simulink model "regcontrol_model"  (Simulink 9.1)
settings: Solver=VariableStepAuto  StartTime=0.0  StopTime=10.0  RelTol=1e-3
values from neighbouring files (symbols this model uses):
  BandWidth = Simulink.Parameter    [start.m]
  BaseVoltage = Simulink.Parameter    [start.m]
  CogenEnabled = false    [regcontrol_emulator.m]    (also in start.m = Simulink.Parameter)
  IsReversible = Simulink.Parameter    [start.m]
  LDC_Z = Simulink.Parameter    [start.m]
  PTratio = Simulink.Parameter    [start.m]
  RevBand = Simulink.Parameter    [start.m]
  RevVreg = Simulink.Parameter    [start.m]
  TapLimitPerChange = Simulink.Parameter    [start.m]
  UsingRegulatedBus = Simulink.Parameter    [start.m]
  Vlimit = Simulink.Parameter    [start.m]
  Vreg = Simulink.Parameter    [start.m]
undefined symbols (not defined in the file or in its folder): ControlModes, m, n
libraries: simulink x3
(part 1 of 2)
settings Model: Creator=Michael Girbino  LastModifiedBy=Michael Girbino
settings DataIOCC: SaveFormat=Dataset
settings OptimizationCC: LifeSpan=auto
settings DebuggingCC: UnderspecifiedInitializationDetection=Simplified  MergeDetectMultiDrivingBlocksExec=error  SFUnexpectedBacktrackingDiag=error  SFNoUnconditionalDefaultTransitionDiag=error  SFExecutionAtInitializationDiag=warning
settings HardwareCC: ProdBitPerPointer=64  ProdBitPerSizeT=64  ProdBitPerPtrDiffT=64  ProdLargestAtomicFloat=Float  ProdIntDivRoundTo=Zero  ProdEndianess=LittleEndian  ProdWordSize=64  ProdHWDeviceType=Intel->x86-64 (Windows64)
settings ModelReferenceCC: PropagateSignalLabelsOutOfModel=on
settings GRTTargetCC: TargetLangStandard=C99 (ISO)  CombineOutputUpdateFcns=on  GRTInterface=off
settings ConfigComp: CovMetricSettings=dwe  CovHtmlReporting=off  CovSaveCumulativeToWorkspaceVar=off  CovSaveSingleToWorkspaceVar=off  CovExternalEMLEnable=on

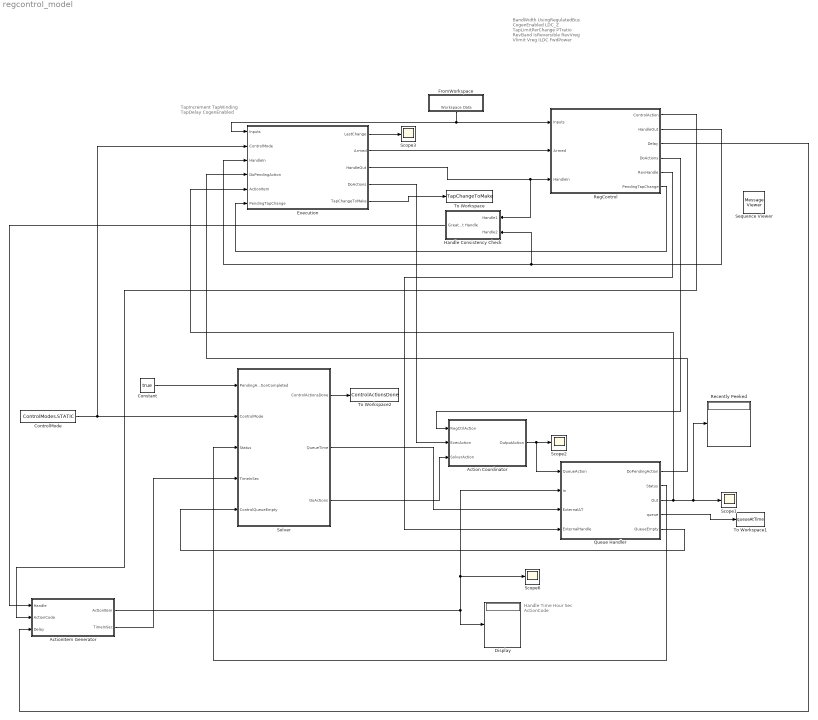
== system regcontrol_model ==
  note: BandWidth
      | UsingRegulatedBus
      | CogenEnabled
      | LDC_Z
      | TapLimitPerChange
      | PTratio
      | RevBand
      | IsReversible
      | RevVreg
      | Vlimit
      | Vreg
      | ILDC
      | FwdPower
  note: Handle
      | Time
      | Hour
      | Sec
      | ActionCode
  note: TapIncrement
      | TapWinding
      | TapDelay
      | CogenEnabled
  Action Coordinator : Stateflow chart  TreatAsAtomicUnit=on
  ActionItem Generator : Subsystem
  Constant : Constant  Value=true  OutDataTypeStr=boolean
  ControlMode : Constant  Value=ControlModes.STATIC  OutDataTypeStr=Enum: ControlModes
  Display : Display
  Execution : Stateflow chart  TreatAsAtomicUnit=on
  FromWorkspace : Subsystem
  Handle Consistency Check : Subsystem
  Queue Handler : Stateflow chart  TreatAsAtomicUnit=on
  Recently Peeked : Display
  RegControl : Stateflow chart  TreatAsAtomicUnit=on
  Scope{1..3,6} (4 alike) : Scope
  Sequence Viewer : MessageViewer
  Solver : Stateflow chart  TreatAsAtomicUnit=on
  To Workspace : ToWorkspace  VariableName=TapChangeToMake  SaveFormat=Timeseries  SampleTime=-1
  To Workspace1 : ToWorkspace  VariableName=queueAtTime  SaveFormat=Structure With Time  SampleTime=-1
  To Workspace2 : ToWorkspace  VariableName=ControlActionsDone  SaveFormat=Timeseries  SampleTime=-1
  wires:
  FromWorkspace/1(Workspace Data) -> Execution/1(Inputs), RegControl/1(Inputs)
  Queue Handler/5(QueueEmpty) -> Solver/5(ControlQueueEmpty)
  Queue Handler/4(queue) -> To Workspace1/1
  Constant/1 -> Solver/1(PendingActionCompleted)
  ActionItem Generator/2(TimeInSec) -> Solver/4(TimeInSec)
  Queue Handler/2(Status) -> Solver/3(Status)
  ControlMode/1 -> Execution/2(ControlMode), Solver/2(ControlMode)
  Solver/2(QueueTime) -> Queue Handler/3(ExternalAT)
  Queue Handler/3(Out) -> Recently Peeked/1, Scope1/1, Execution/5(ActionItem)
  ActionItem Generator/1(ActionItem) -> Scope6/1, Queue Handler/2(In), Display/1
  Solver/1(ControlActionsDone) -> To Workspace2/1
  RegControl/1(ControlAction) -> ActionItem Generator/2(ActionCode)
  Action Coordinator/1(OutputAction) -> Queue Handler/1(QueueAction), Scope2/1
  Solver/3(DoActions) -> Action Coordinator/3(SolverAction)
  Execution/4(DoActions) -> Action Coordinator/2(ExecAction)
  RegControl/4(DoActions) -> Action Coordinator/1(RegCtrlAction)
  RegControl/3(Delay) -> ActionItem Generator/3(Delay)
  RegControl/2(HandleOut) -> Handle Consistency Check/2(Handle2), Execution/3(HandleIn)
  RegControl/5(RevHandle) -> Queue Handler/4(ExternalHandle)
  Execution/3(HandleOut) -> Handle Consistency Check/1(Handle1), RegControl/3(HandleIn)
  Execution/2(Armed) -> RegControl/2(Armed)
  Queue Handler/1(DoPendingAction) -> Execution/4(DoPendingAction)
  Execution/5(TapChangeToMake) -> To Workspace/1
  RegControl/6(PendingTapChange) -> Execution/6(PendingTapChange)
  Execution/1(LastChange) -> Scope3/1
  Handle Consistency Check/1(Greatest Handle) -> ActionItem Generator/1(Handle)

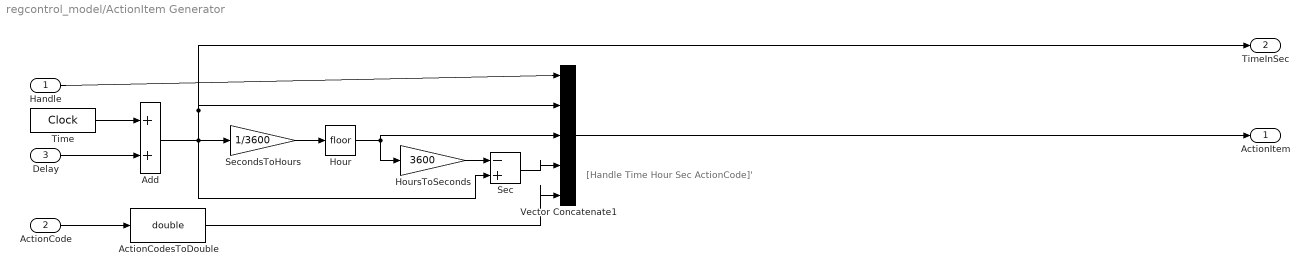
== system regcontrol_model/ActionItem Generator ==
  note: [Handle Time Hour Sec ActionCode]'
  Handle : Inport
  ActionCode : Inport  Port=2
  Delay : Inport  Port=3
  ActionCodesToDouble : DataTypeConversion  OutDataTypeStr=double
  Add : Sum
  Hour : Rounding
  HoursToSeconds : Gain  Gain=3600
  Sec : Sum  Inputs=-+
  SecondsToHours : Gain  Gain=1/3600
  Time : DigitalClock
  Vector Concatenate1 : Concatenate  NumInputs=5
  ActionItem : Outport
  TimeInSec : Outport  Port=2
  wires:
  Add/1 -> Sec/2, SecondsToHours/1, TimeInSec/1, Vector Concatenate1/2
  Hour/1 -> Vector Concatenate1/3, HoursToSeconds/1
  SecondsToHours/1 -> Hour/1
  Vector Concatenate1/1 -> ActionItem/1
  HoursToSeconds/1 -> Sec/1
  Handle/1 -> Vector Concatenate1/1
  Sec/1 -> Vector Concatenate1/4
  Delay/1 -> Add/2
  Time/1 -> Add/1
  ActionCode/1 -> ActionCodesToDouble/1
  ActionCodesToDouble/1 -> Vector Concatenate1/5

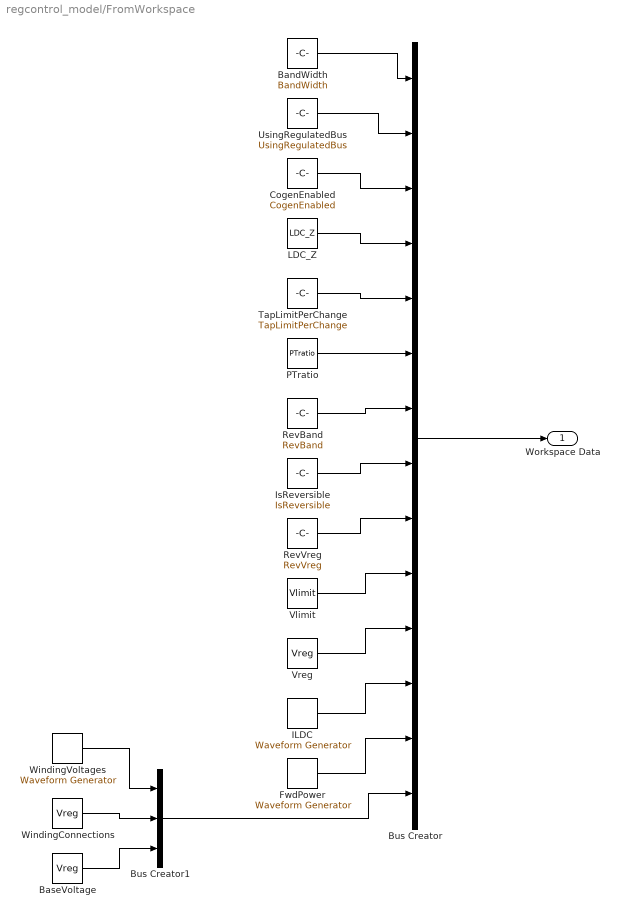
== system regcontrol_model/FromWorkspace ==
  BandWidth : Constant  Value=BandWidth
  BaseVoltage : Constant  Value=Vreg
  Bus Creator : BusCreator  Inputs=14  OutDataTypeStr=Bus: InputsBus
  Bus Creator1 : BusCreator  Inputs=3  OutDataTypeStr=Bus: ControlledTransformer
  CogenEnabled : Constant  Value=CogenEnabled
  FwdPower : simulink/Sources/Waveform Generator  OutMin=[]  OutMax=[]  OutDataTypeStr=double  SelectedSignal=1  Signals=FwdPower  BlockNames=MultiportSwitch_38ca288ec892465  SampleTime=0.1
      settings: SourceProductName=Simulink
  ILDC : simulink/Sources/Waveform Generator  OutMin=[]  OutMax=[]  OutDataTypeStr=double  SelectedSignal=1  Signals=ILDC  BlockNames=MultiportSwitch_5ceb58a2c9c749f  SampleTime=0.1
      settings: SourceProductName=Simulink
  IsReversible : Constant  Value=IsReversible
  LDC_Z : Constant  Value=LDC_Z
  PTratio : Constant  Value=PTratio
  RevBand : Constant  Value=RevBand
  RevVreg : Constant  Value=RevVreg
  TapLimitPerChange : Constant  Value=TapLimitPerChange
  UsingRegulatedBus : Constant  Value=UsingRegulatedBus
  Vlimit : Constant  Value=Vlimit
  Vreg : Constant  Value=Vreg
  WindingConnections : Constant  Value=Vreg
  WindingVoltages : simulink/Sources/Waveform Generator  OutMin=[]  OutMax=[]  OutDataTypeStr=double  SelectedSignal=1  Signals=FwdPower  BlockNames=MultiportSwitch_38ca288ec892465  SampleTime=0.1
      settings: SourceProductName=Simulink
  Workspace Data : Outport
  wires:
  ILDC/1 -> Bus Creator/12
  Vlimit/1 -> Bus Creator/10
  LDC_Z/1 -> Bus Creator/4
  BandWidth/1 -> Bus Creator/1
  TapLimitPerChange/1 -> Bus Creator/5
  FwdPower/1 -> Bus Creator/13
  PTratio/1 -> Bus Creator/6
  Vreg/1 -> Bus Creator/11
  IsReversible/1 -> Bus Creator/8
  RevVreg/1 -> Bus Creator/9
  Bus Creator/1 -> Workspace Data/1
  RevBand/1 -> Bus Creator/7
  UsingRegulatedBus/1 -> Bus Creator/2
  CogenEnabled/1 -> Bus Creator/3
  Bus Creator1/1 -> Bus Creator/14
  WindingVoltages/1 -> Bus Creator1/1
  WindingConnections/1 -> Bus Creator1/2
  BaseVoltage/1 -> Bus Creator1/3

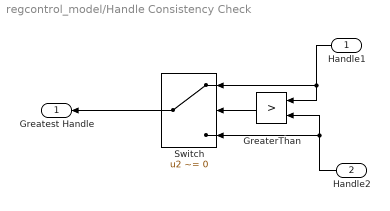
== system regcontrol_model/Handle Consistency Check ==
  Handle1 : Inport
  Handle2 : Inport  Port=2
  GreaterThan : RelationalOperator  Operator=>  RndMeth=Simplest
  Switch : Switch  Criteria=u2 ~= 0
  Greatest Handle : Outport
  wires:
  Handle2/1 -> GreaterThan/2, Switch/3
  GreaterThan/1 -> Switch/2
  Handle1/1 -> GreaterThan/1, Switch/1
  Switch/1 -> Greatest Handle/1

== stateflow chart Execution ==
  settings: executeAtInitialization=1
  state Push(CodeVal, DelayVal) [function]
    (default) -> (junction 24) : {ActionCode = CodeVal;
        | Delay = DelayVal;
        | HandleOut = HandleOut + 1;
        | DoActions.data = QueueActions.PUSH;
        | send(DoActions);}
  state AssignInputsToLocals [function]
    (default) -> (junction 26) : {% From Script:
        | TapIncrement = Inputs.TapIncrementl
        | TapWinding = Inputs.TapWinding;
        | TapDelay = Inputs.TapDelay;
        | CogenEnabled = Inputs.CogenEnabled;
        | % From the ControlQueue:
        | Code = ...
        | ActionItem(NewControlQueueFields.ActionCode);
        | % PendingTapChange:
        | LocalPendingTapChange = PendingTapChange;}
    (junction 26) -> (junction 27) [order 1] : [HandleIn > HandleOut]
    (junction 26) -> (junction 28) [order 2]
    (junction 27) -> (junction 29) : {HandleOut = HandleIn;}
    (junction 29) -> (junction 28)
    (junction 28) -> (junction 30)
  state ChangeToMake = AtLeastOneTap(ProposedChange, Increment) [function]
    note: Called in STATIC mode
        | Changes 70% of the way but at least one tap, subject to maximum allowable tap change
    (default) -> (junction 40) : {NumTaps = floor(0.7 * abs(ProposedChange)/Increment);}
    (junction 40) -> (junction 41) [order 1] : [NumTaps == 0]
    (junction 40) -> (junction 42) [order 2]
    (junction 41) -> (junction 43) : {NumTaps = 1;} % At least 1 tap
    (junction 43) -> (junction 42)
    (junction 42) -> (junction 44)
    (junction 44) -> (junction 45) [order 1] : [NumTaps > TapLimitPerChange]
    (junction 44) -> (junction 46) [order 2]
    (junction 45) -> (junction 47) : {NumTaps = TapLimitPerChange;} % Bound by maximum
    (junction 47) -> (junction 46)
    (junction 46) -> (junction 48) : {LastChange = NumTaps;}
    (junction 48) -> (junction 49) [order 1] : % Check sign on change:
        | [ProposedChange > 0]
    (junction 48) -> (junction 50) [order 2] : {ChangeToMake = -1*NumTaps*Increment;
        | LastChange = -1*NumTaps;}
    (junction 49) -> (junction 51) : {ChangeToMake =...
        |  NumTaps*Increment;}
    (junction 51) -> (junction 50)
    (junction 50) -> (junction 52)
  state [ChangeToMake, NewProposedChange] = OneInDirectionOf(ProposedChange, Increment) [function]
    note: Computes the amount of one tap change in the direction of the pending tapchange
        | Automatically decrements the proposed change by that amount
    (default) -> (junction 103) : {LastChange = 0;}
    (junction 103) -> (junction 104) [order 1] : [ProposedChange > 0]
    (junction 103) -> (junction 105) [order 2] : {ChangeToMake = -1*Increment;
        | LastChange = -1;
        | NewProposedChange = ProposedChange + Increment;}
    (junction 104) -> (junction 106) : {ChangeToMake = Increment;
        | LastChange = 1;
        | NewProposedChange =...
        |  ProposedChange - Increment;}
    (junction 106) -> (junction 105)
    (junction 105) -> (junction 107)
    (junction 107) -> (junction 108) [order 1] : [abs(NewProposedChange) < 0.9*Increment]
    (junction 107) -> (junction 109) [order 2]
    (junction 108) -> (junction 110) : {NewProposedChange = 0;}
    (junction 110) -> (junction 109)
    (junction 109) -> (junction 111)
  state ResetTransitionFlags [function]
    (default) -> (junction 132) : {EXIT_TAPCHANGE = false;
        | EXIT_REVERSE = false;}
  state ControlFlow
    state Finished
    state Reversing
      state FlipReverse
        (default) -> (junction 90)
        (junction 90) -> (junction 91) [order 1] : [InReverseMode]
        (junction 90) -> (junction 92) [order 2] : {InReverseMode = true;}
        (junction 91) -> (junction 93) : {InReverseMode = false;}
        (junction 93) -> (junction 92)
      state FlipCogen
        (default) -> (junction 123)
        (junction 123) -> (junction 124) [order 1] : [InCogenMode]
        (junction 123) -> (junction 125) [order 2] : {InCogenMode = true;}
        (junction 124) -> (junction 126) : {InCogenMode = false;}
        (junction 126) -> (junction 125)
      state Finished
        en: EXIT_REVERSE = true;
      (default) -> (junction 69)
      (junction 69) -> (junction 70) [order 1] : [ReversePending]
      (junction 69) -> (junction 75) [order 2]
      (junction 70) -> (junction 71)
      (junction 71) -> (junction 72) [order 1] : [CogenEnabled]
      (junction 71) -> FlipReverse [order 2]
      (junction 72) -> FlipCogen : % Cogen mode takes precedence if present
      FlipCogen -> (junction 74)
      FlipReverse -> (junction 73)
      (junction 74) -> (junction 73)
      (junction 73) -> (junction 76) : {ReversePending = false;}
      (junction 76) -> (junction 75)
      (junction 75) -> ControlFlow.Reversing.Finished
    state MakingTapChange
      state Finished
        en: EXIT_TAPCHANGE = true;
      state StaticTapChange
        (default) -> (junction 193) : {TapChangeToMake = AtLeastOneTap(PendingTapChange, TapIncrement(TapWinding));
            | % reset to no change = change - 1 program will determin if another is needed:
            | PendingTapChange = 0;
            | Armed = false;}
      state EventDrivenTapChange
        (default) -> (junction 195) : {[TapChangeToMake LocalPendingTapChange] =...
            |  OneInDirectionOf(LocalPendingTapChange, TapIncrement(TapWinding));
            | PresentTap(TapWinding) = PresentTap(TapWinding) + TapChangeToMake;}
        (junction 195) -> (junction 196) [order 1] : [PendingTapChange ~= 0]
        (junction 195) -> (junction 197) [order 2] : {Armed = false;}
        (junction 196) -> (junction 198) : {Push(ActionCodes.ACTION_TAPCHANGE, TapDelay);}
        (junction 198) -> (junction 197)
      state TimeDrivenTapChange
        (default) -> (junction 204) : {[TapChangeToMake LocalPendingTapChange] =...
            |  OneInDirectionOf(LocalPendingTapChange, TapIncrement(TapWinding));
            | PresentTap(TapWinding) = PresentTap(TapWinding) + TapChangeToMake;}
        (junction 204) -> (junction 205) [order 1] : [PendingTapChange ~= 0]
        (junction 204) -> (junction 206) [order 2] : {Armed = false;}
        (junction 205) -> (junction 207) : {Push(ActionCodes.ACTION_TAPCHANGE, TapDelay);}
        (junction 207) -> (junction 206)
      state MultiRateTapChange
        (default) -> (junction 213) : {[TapChangeToMake LocalPendingTapChange] =...
            |  OneInDirectionOf(LocalPendingTapChange, TapIncrement(TapWinding));
            | PresentTap(TapWinding) = PresentTap(TapWinding) + TapChangeToMake;}
        (junction 213) -> (junction 214) [order 1] : [PendingTapChange ~= 0]
        (junction 213) -> (junction 215) [order 2] : {Armed = false;}
        (junction 214) -> (junction 216) : {Push(ActionCodes.ACTION_TAPCHANGE, TapDelay);}
        (junction 216) -> (junction 215)
      (default) -> (junction 153)
      (junction 153) -> (junction 154) [order 1] : % Check to make sure control has not reset:
          | [PendingTapChange == 0]
      (junction 153) -> (junction 155) [order 2]
      (junction 154) -> (junction 167) : {Armed = false;}
      (junction 155) -> StaticTapChange [order 1] : [ControlMode == ControlModes.STATIC]
      (junction 155) -> (junction 156) [order 2]
      StaticTapChange -> (junction 158)
      (junction 156) -> EventDrivenTapChange [order 1] : [ControlMode == ControlModes.EVENTDRIVEN]
      (junction 156) -> (junction 159) [order 2]
      EventDrivenTapChange -> (junction 157)
      (junction 157) -> (junction 158)
      (junction 158) -> (junction 161)
      (junction 159) -> TimeDrivenTapChange [order 1] : [ControlMode == ControlModes.TIMEDRIVEN]
      (junction 159) -> (junction 162) [order 2]
      TimeDrivenTapChange -> (junction 160)
      (junction 160) -> (junction 161)
      (junction 161) -> (junction 163)
      (junction 162) -> MultiRateTapChange [order 1] : [ControlMode == ControlModes.MULTIRATE]
      (junction 162) -> (junction 164) [order 2]
      (junction 163) -> (junction 166)
      MultiRateTapChange -> (junction 165)
      (junction 165) -> (junction 164)
      (junction 166) -> (junction 165)
      (junction 164) -> ControlFlow.MakingTapChange.Finished
      (junction 167) -> ControlFlow.MakingTapChange.Finished
    (default) -> (junction 134) : {AssignInputsToLocals();
        | ResetTransitionFlags();}
    (junction 134) -> MakingTapChange [order 1] : [Code == ActionCodes.ACTION_TAPCHANGE]
    (junction 134) -> (junction 137) [order 2]
    MakingTapChange -> (junction 135) : [EXIT_TAPCHANGE]
    (junction 135) -> (junction 136)
    (junction 136) -> (junction 138)
    (junction 137) -> Reversing [order 1] : [Code == ActionCodes.ACTION_REVERSE]
    (junction 137) -> (junction 139) [order 2]
    Reversing -> (junction 138)
    (junction 138) -> (junction 140) : [EXIT_REVERSE]
    (junction 140) -> (junction 139)
    (junction 139) -> ControlFlow.Finished
  (default) -> ControlFlow : DoPendingAction
  data: CodeVal function_input double; DelayVal function_input double; ProposedChange function_input double; Increment function_input double; ChangeToMake function_output double; ProposedChange function_input double; Increment function_input double; ChangeToMake function_output double; NewProposedChange function_output double; Inputs input Bus: InputsBus; LastChange output double; Change local double; NumTaps local uint8; ControlMode input Enum: ControlModes; HandleIn input double; Armed output boolean; HandleOut output double =0; DoActions output boolean =false; PresentTap local uint8; EXIT_REVERSE local boolean; InReverseMode local boolean; EXIT_TAPCHANGE local boolean; ReversePending local boolean; InCogenMode local boolean; DoPendingAction input boolean; TapWinding local uint8; TapIncrement local double; TapDelay local double; CogenEnabled local boolean =false; Code local Enum: ActionCodes; ActionItem input double size=[1 5]; TapChangeToMake output double; PendingTapChange input double; LocalPendingTapChange local double

== stateflow chart Solver ==
  state ControlFlow
    note: Static
        | - placeholder QueueTime
        | - DoNearestActions
    note: Event-driven
        | - QueueTime is current time
        | - DoNearestActions
    note: Time-driven
        | - QueueTime is current time
        | - DoActions
    note: Multirate
        | - QueueTime is current time
        | - DoMultiRate
    (default) -> (junction 256)
    (junction 256) -> (junction 257) [order 1] : [ControlMode == ControlModes.STATIC]
    (junction 256) -> (junction 264) [order 2]
    (junction 257) -> (junction 258)
    (junction 258) -> (junction 259) [order 1] : [LocalControlQueueEmpty]
        | % execute nearest set of control actions, but leave time where it is
    (junction 258) -> (junction 260) [order 2] : {QueueTime = 0; %[0 0] xHour, xSec
        | DoActions.data = QueueActions.DO_NEAREST_ACTIONS;
        | send(DoActions);
        | % ignores time advancement
        | }
    (junction 259) -> (junction 261) : {ControlActionsDone = true;}
    (junction 261) -> (junction 260)
    (junction 260) -> (junction 262)
    (junction 262) -> (junction 263)
    (junction 263) -> (junction 271)
    (junction 264) -> (junction 265) [order 1] : [ControlMode == ControlModes.EVENTDRIVEN]
        | % execute nearest set of control actions and advance time to that time
    (junction 265) -> (junction 266) : {QueueTime = TimeInSec; %xHour, xSec
        | DoActions.data = QueueActions.DO_NEAREST_ACTIONS;
        | send(DoActions);}
    (junction 264) -> (junction 272) [order 2]
    (junction 266) -> (junction 267) [order 1] : [~PendingActionCompleted]
    (junction 266) -> (junction 268) [order 2]
    (junction 267) -> (junction 269) : {ControlActionsDone = true;
        | % advances time to the next event
        | }
    (junction 269) -> (junction 268)
    (junction 268) -> (junction 270)
    (junction 270) -> (junction 271)
    (junction 271) -> (junction 279)
    (junction 272) -> (junction 273) [order 1] : [ControlMode == ControlModes.TIMEDRIVEN]
        |  % Do all actions having and action time <= specified time
    (junction 272) -> (junction 280) [order 2]
    (junction 273) -> (junction 274) : {QueueTime = TimeInSec; %xHour, xSec
        | DoActions.data = QueueActions.DO_ACTIONS;
        | send(DoActions);}
    (junction 274) -> (junction 275) [order 1] : [~PendingActionCompleted]
    (junction 274) -> (junction 276) [order 2]
    (junction 275) -> (junction 277) : {ControlActionsDone = true;
        | }
    (junction 277) -> (junction 276)
    (junction 276) -> (junction 278)
    (junction 278) -> (junction 279)
    (junction 279) -> (junction 287)
    (junction 280) -> (junction 281) [order 1] : [ControlMode == ControlModes.MULTIRATE]
        |  % Execute the nearest set of control actions, but leave time where it is
    (junction 280) -> (junction 288) [order 2]
    (junction 281) -> (junction 282) : {QueueTime =TimeInSec; %xHour, xSec
        | DoActions.data = QueueActions.DO_MULTIRATE;
        | send(DoActions);}
    (junction 282) -> (junction 283) [order 1] : [~PendingActionCompleted]
    (junction 282) -> (junction 284) [order 2]
    (junction 283) -> (junction 285) : {ControlActionsDone = true;
        | }
    (junction 285) -> (junction 284)
    (junction 284) -> (junction 286)
    (junction 286) -> (junction 287)
    (junction 287) -> (junction 289)
    (junction 289) -> (junction 288)
    (junction 288) -> (junction 290)
  state QueueEmptyCase
    en: LocalControlQueueEmpty = true;
  (default) -> ControlFlow
  QueueEmptyCase -> ControlFlow
  ControlFlow -> QueueEmptyCase : ControlQueueEmpty
  data: ControlActionsDone output boolean; QueueTime output double; DoActions output Enum: QueueActions; PendingActionCompleted input boolean; ControlMode input Enum: ControlModes; ii local double =0; Status input Enum: Statuses; TimeInSec input double; LocalControlQueueEmpty local boolean =false; ControlQueueEmpty input boolean

== stateflow chart RegControl ==
  settings: executeAtInitialization=1
  state ControlFlow
    state DetermineReversePendingLookingForward
      state CorrectFalseReversePending
        (default) -> (junction 461)
        (junction 461) -> (junction 462) [order 1] : [FwdPower < (-1*RevPowerThreshold)]
        (junction 461) -> (junction 463) [order 2]
        (junction 462) -> (junction 464) : {ReversePending = true;
            | RevHandle = ...
            | Push(ActionCodes.ACTION_REVERSE, ...
            | RevDelay);
            | }
        (junction 464) -> (junction 463)
      state CorrectTrueReversePending
        (default) -> (junction 471)
        (junction 471) -> (junction 470) [order 1] : [FwdPower >= (-1*RevPowerThreshold)]
        (junction 471) -> (junction 472) [order 2]
        (junction 470) -> (junction 473) : % Reset ReversePending:
            | % Delete RevHandle from ControlQueue
            | {DoActions.data = QueueActions.DELETE;
            | send(DoActions);
            | ReversePending = false;
            | RevHandle = 0;}
        (junction 473) -> (junction 472)
      state Finished
        en: GET_VOLTAGE = true;
      (default) -> (junction 448) : {FwdPower = -1*real( ControlledTransformer.Power(ElementTerminal) );}
          | % Should we reverse?
      (junction 448) -> ControlFlow.DetermineReversePendingLookingForward.CorrectFalseReversePending [order 1] : [~ReversePending]
      (junction 448) -> (junction 449) [order 2]
      ControlFlow.DetermineReversePendingLookingForward.CorrectFalseReversePending -> (junction 449)
      (junction 449) -> (junction 450)
      (junction 450) -> ControlFlow.DetermineReversePendingLookingForward.CorrectTrueReversePending [order 1] : [ReversePending]
      (junction 450) -> (junction 451) [order 2]
      ControlFlow.DetermineReversePendingLookingForward.CorrectTrueReversePending -> (junction 451)
      (junction 451) -> ControlFlow.DetermineReversePendingLookingForward.Finished
    state DetermineReversePendingLookingReverseOrCogen
      state CorrectFalseReversePending
        (default) -> (junction 492)
        (junction 492) -> (junction 493) [order 1] : [FwdPower > RevPowerThreshold]
        (junction 492) -> (junction 494) [order 2]
        (junction 493) -> (junction 495) : {ReversePending = true;
            | RevHandle = ...
            | Push(ActionCodes.ACTION_REVERSE, ...
            | RevDelay);
            | }
        (junction 495) -> (junction 494)
      state CorrectTrueReversePending
        (default) -> (junction 501)
        (junction 501) -> (junction 502) [order 1] : [FwdPower <= RevPowerThreshold]
        (junction 501) -> (junction 503) [order 2]
        (junction 502) -> (junction 504) : % Reset ReversePending:
            | {ReversePending = false;}
        (junction 504) -> (junction 503)
      state Finished
        en: REV_NEUTRAL = true;
      (default) -> (junction 479) : {FwdPower = -1*real( ControlledTransformer.Power(ElementTerminal) );}
          | % If reversed, check if power is back in forward direction
      (junction 479) -> ControlFlow.DetermineReversePendingLookingReverseOrCogen.CorrectFalseReversePending [order 1] : [~ReversePending]
      (junction 479) -> (junction 480) [order 2]
      ControlFlow.DetermineReversePendingLookingReverseOrCogen.CorrectFalseReversePending -> (junction 480)
      (junction 480) -> (junction 481)
      (junction 481) -> ControlFlow.DetermineReversePendingLookingReverseOrCogen.CorrectTrueReversePending [order 1] : [ReversePending]
      (junction 481) -> (junction 482) [order 2]
      ControlFlow.DetermineReversePendingLookingReverseOrCogen.CorrectTrueReversePending -> (junction 482)
      (junction 482) -> ControlFlow.DetermineReversePendingLookingReverseOrCogen.Finished
    state ReverseNeutralCase
      state Finished
        send(GET_VOLTAGE);
      state Exiting
        en: EXIT = true;
      (default) -> (junction 510)
      (junction 510) -> (junction 511) [order 1] : % tap change not specified as needed:
          | [~Armed]
      (junction 510) -> ControlFlow.ReverseNeutralCase.Finished [order 2]
      (junction 511) -> (junction 512) : {PendingTapChange = 0.0;}
      (junction 512) -> (junction 513) [order 1] : [abs(PresentTap(TapWinding) - 1.0) < EPSILON]
      (junction 512) -> Exiting [order 2]
      (junction 513) -> (junction 514) : {Increment = TapIncrement(TapWinding);
          | PendingTapChange = round( (1.0 - ...
          | PresentTap(TapWinding)) / Increment ) * Increment;}
      (junction 514) -> (junction 515) [order 1] : [PendingTapChange ~= 0.0 && ~Armed]
      (junction 515) -> (junction 517) : {% Push ACTION_TAPCHANGE
          | % to ControlQueue with TapDelay:
          | Push(ActionCodes.ACTION_TAPCHANGE, TapDelay);
          | Armed = true;}
      (junction 514) -> (junction 516) [order 2]
      (junction 517) -> (junction 516)
      (junction 516) -> (junction 518)
      (junction 518) -> Exiting
    state GetVoltage
      state Finished
        en: DETERMINE_VLOCALBUS = true;
      (default) -> (junction 532)
      (junction 532) -> (junction 533) [order 1] : [UsingRegulatedBus]
      (junction 532) -> ControlFlow.GetVoltage.Finished [order 2] : {VBuffer = ControlledTransformerWindingVoltages;
          | %ControlledTransformer.GetWindingVoltages;
          | Vcontrol = GetControlVoltage(VBuffer, Fnphases, PTRatio);}
      (junction 533) -> (junction 534) : {TransformerConnection = ControlledTransformerConnection;
          | %TransformerConnection = ControlledTransformer.Winding(ElementTerminal).Connection;
          | Vterminal = ComputeVTerminal(NodeV);}
      (junction 534) -> ControlFlow.GetVoltage.Finished
    state DetermineVlocalbus
      state Finished
        en: GET_VOLTAGEWLDC = true;
      (default) -> (junction 540)
      (junction 540) -> (junction 541) [order 1] : % Voltage limit for bus connected to regulated winding; default = 0.0 (inactive)
          | [VlimitActive]
      (junction 540) -> ControlFlow.DetermineVlocalbus.Finished [order 2] : {Vlocalbus = 0.0;}
      (junction 541) -> (junction 542)
      (junction 542) -> (junction 543) [order 1] : % when controlled transformer is different from LDC PTransformer
          | [UsingRegulatedBus]
      (junction 542) -> (junction 544) [order 2] : % controlled transformer is
          | % the LDC PTransformer
          | {Vlocalbus = abs(Vcontrol);}
      (junction 543) -> (junction 545) : {ControlledTransformer.GetWindingVoltages(ElementTerminal, VBuffer);
          | Vlocalbus = abs( VBuffer(1) / PTRatio );}
      (junction 545) -> (junction 544)
      (junction 544) -> (junction 546)
      (junction 546) -> ControlFlow.DetermineVlocalbus.Finished
    state GetVoltageWithLDC
      state RX_LDCmode
        (default) -> (junction 563)
        (junction 563) -> (junction 564) [order 1] : [InReverseMode || InCogenMode]
        (junction 563) -> (junction 565) [order 2] : {VLDC = complex(R, X) * complex( real(ILDC), imag(ILDC) );}
        (junction 564) -> (junction 566) : {VLDC = complex(revR, revX) * complex( real(ILDC), imag(ILDC) );}
        (junction 566) -> (junction 565)
      state Z_LDCmode
        (default) -> (junction 572)
        (junction 572) -> (junction 573) [order 1] : [InReverseMode || InCogenMode]
        (junction 572) -> (junction 574) [order 2] : {Vcontrol = abs(Vcontrol) - abs(ILDC) * LDC_Z;}
        (junction 573) -> (junction 575) : {Vcontrol = abs(Vcontrol) - abs(ILDC) * revLDC_Z;}
        (junction 575) -> (junction 574)
      state Finished
        en: GET_TEST_VALUES = true;
      (default) -> (junction 557) : {ControlledElement.GetCurrents(CBuffer);
          | %Convert current to control current by CTRating:
          | ILDC = CBuffer( ControlledElement.Nconds * (ElementTerminal - 1) + ControlledPhase);}
      (junction 557) -> RX_LDCmode [order 1] : % Standard R, X LDC
          | [LDC_Z == 0.0]
      (junction 557) -> Z_LDCmode [order 2] : % Beckwith LDC_Z control mode
      Z_LDCmode -> ControlFlow.GetVoltageWithLDC.Finished
      RX_LDCmode -> ControlFlow.GetVoltageWithLDC.Finished
    state GetTestValues
      state Finished
        en:
        DETERMINE_TAP_CHANGE = true;
      (default) -> (junction 581) : % assumes looking forward:
          | {Vactual = abs(Vcontrol);}
      (junction 581) -> (junction 582) [order 1] : [InReverseMode]
      (junction 581) -> ControlFlow.GetTestValues.Finished [order 2] : {VregTest = Vreg;
          | BandTest = Bandwidth;}
      (junction 582) -> (junction 583) : {Vactual = Vactual / PresentTap(Winding);
          | VregTest = RevVreg;
          | BandTest = RevBandwidth;}
      (junction 583) -> ControlFlow.GetTestValues.Finished
    state DetermineTapChangeIsNeeded
      state Finished
        en:
        MAKE_TAP_CHANGE = true;
      (default) -> (junction 589)
      (junction 589) -> (junction 590) [order 1] : % difference between desired and actual > half bandwidth
          | [abs(VregTest - Vactual) > BandTest/2.0]
      (junction 589) -> ControlFlow.DetermineTapChangeIsNeeded.Finished [order 2] : {TapChangeIsNeeded = false;}
      (junction 590) -> (junction 591) : {TapChangeIsNeeded = true;}
      (junction 591) -> ControlFlow.DetermineTapChangeIsNeeded.Finished
    state MakeTapChange
      state GetVboostFromVlimit
        (default) -> (junction 626)
        (junction 626) -> (junction 627) [order 1] : [Vlocalbus > Vlimit]
        (junction 626) -> (junction 628) [order 2]
        (junction 627) -> (junction 629) : {Vboost = Vlimit - Vlocalbus;}
        (junction 629) -> (junction 628)
      state TapChangeUp
        (default) -> (junction 635)
        (junction 635) -> (junction 636) [order 1] : [PresentTap(TapWinding) < MaxTap(TapWinding)]
        (junction 635) -> (junction 637) [order 2]
        (junction 636) -> (junction 638) : {% push ACTION_TAPCHANGE to ControlQueue
            | % with delay ComputeTimeDelay(Vactual):
            | Push(ActionCodes.ACTION_TAPCHANGE, ...
            | ComputeTimeDelay(Vactual));
            | Armed = true;}
        (junction 638) -> (junction 637)
      state TapChangeDown
        (default) -> (junction 644) : % going down:
        (junction 644) -> (junction 645) [order 1] : [PresentTap(TapWinding) > MinTap(TapWinding)]
        (junction 644) -> (junction 646) [order 2]
        (junction 645) -> (junction 647) : {% push ACTION_TAPCHANGE to ControlQueue
            | % with delay ComputeTimeDelay(Vactual):
            | Push(ActionCodes.ACTION_TAPCHANGE, ...
            | ComputeTimeDelay(Vactual));
            | Armed = true;}
        (junction 647) -> (junction 646)
      state Finished
        en: FINISHED = true;
      (default) -> (junction 597) : % compute tapchange:
          | {Vboost = VregTest - Vactual;}
      (junction 597) -> (junction 598) [order 1] : [VlimitActive]
      (junction 597) -> (junction 599) [order 2]
      (junction 598) -> GetVboostFromVlimit
      GetVboostFromVlimit -> (junction 600)
      (junction 600) -> (junction 599)
      (junction 599) -> (junction 601) : {% PU winding boost needed:
          | BoostNeeded = Vboost * PTRatio / BaseVoltage(ElementTerminal);
          | Increment = TapIncrement(TapWinding);
          | % quantize to an increment:
          | PendingTapChange = round(BoostNeeded/Increment)*Increment;}
      (junction 601) -> (junction 602) : % send initial tap change message to ControlQueue, add delay time to solution control queue:
      (junction 602) -> (junction 603) [order 1] : % only changes 1 tap at a time:
          | [PendingTapChange ~= 0.0 && ~Armed]
      (junction 602) -> ControlFlow.MakeTapChange.Finished [order 2]
      (junction 603) -> (junction 604) : % see of any tap change is possible in desired direction (not saturated):
      (junction 604) -> TapChangeUp [order 1] : % going up:
          | [PendingTapChange > 0.0]
      (junction 604) -> TapChangeDown [order 2]
      TapChangeUp -> (junction 606)
      TapChangeDown -> (junction 605)
      (junction 606) -> (junction 605)
      (junction 605) -> (junction 607)
      (junction 607) -> ControlFlow.MakeTapChange.Finished
    state Finished
    (default) -> (junction 386) : {AssignInputsToLocals();
        | ResetTransitionFlags();}
    (junction 386) -> (junction 387) [order 2]
    (junction 387) -> (junction 388)
    (junction 386) -> (junction 399) [order 1] : [TapLimitPerChange == 0]
    (junction 388) -> (junction 389) [order 1] : [~UsingRegulatedBus]
    (junction 389) -> (junction 390)
    (junction 388) -> (junction 395) [order 2]
    (junction 390) -> (junction 391) [order 1] : [IsReversible || CogenEnabled]
    (junction 390) -> (junction 396) [order 2]
    (junction 391) -> (junction 392)
    (junction 392) -> DetermineReversePendingLookingForward [order 1] : [LookingForward && ~InCogenMode]
    (junction 392) -> DetermineReversePendingLookingReverseOrCogen [order 2]
    DetermineReversePendingLookingForward -> (junction 398) : [GET_VOLTAGE]
    DetermineReversePendingLookingReverseOrCogen -> (junction 393) : [REV_NEUTRAL]
    (junction 393) -> ReverseNeutralCase [order 1] : % mode for which tap change may be executed,
        | % but no reversal made:
        | [ReverseNeutral]
    (junction 393) -> (junction 394) [order 2]
    ReverseNeutralCase -> (junction 394) [order 2] : GET_VOLTAGE
    (junction 394) -> (junction 397)
    ReverseNeutralCase -> (junction 400) [order 1] : [EXIT]
    (junction 396) -> (junction 395)
    (junction 397) -> (junction 396)
    (junction 398) -> (junction 397)
    (junction 395) -> GetVoltage
    (junction 400) -> (junction 399)
    (junction 399) -> (junction 407)
    GetVoltage -> DetermineVlocalbus : [DETERMINE_VLOCALBUS]
    DetermineVlocalbus -> (junction 401) : [GET_VOLTAGEWLDC]
    (junction 401) -> GetVoltageWithLDC [order 1] : % line drop compensation, but not using regulated bus
        | [~UsingRegulatedBus && LDCActive]
    (junction 401) -> (junction 402) [order 2]
    GetVoltageWithLDC -> (junction 403) : [GET_TEST_VALUES]
    (junction 403) -> (junction 402)
    (junction 402) -> GetTestValues
    GetTestValues -> DetermineTapChangeIsNeeded : [DETERMINE_TAP_CHANGE]
    DetermineTapChangeIsNeeded -> (junction 404) : [MAKE_TAP_CHANGE]
    (junction 404) -> MakeTapChange [order 1] : [TapChangeIsNeeded]
    (junction 404) -> (junction 405) [order 2]
    MakeTapChange -> (junction 406) : [FINISHED]
    (junction 406) -> (junction 405)
    (junction 405) -> ControlFlow.Finished
    (junction 407) -> ControlFlow.Finished : {PendingTapChange = 0;}
  state h = Push(CodeVal, DelayVal) [function]
    (default) -> (junction 656) : {ActionCode = CodeVal;
        | Delay = DelayVal;
        | HandleOut = HandleOut + 1;
        | DoActions.data = QueueActions.PUSH;
        | send(DoActions);
        | h = HandleOut;}
  state AssignInputsToLocals [function]
    (default) -> (junction 658) : {BandWidth = Inputs.Bandwidth;
        | UsingRegulatedBus = Inputs.UsingRegulatedBus;
        | CogenEnabled = Inputs.CogenEnabled;
        | LDC_Z = Inputs.LDC_Z;
        | TapLimitPerChange = Inputs.TapLimitPerChange;
        | PTratio = Inputs.PTratio;
        | RevBand = Inputs.RevBand;
        | IsReversible = Inputs.IsReversible;
        | RevVreg = Inputs.RevVreg;
        | Vlimit = Inputs.Vlimit;
        | Vreg = Inputs.Vreg;
        | ILDC = Inputs.ILDC;
        | FwdPower = Inputs.FwdPower;}
    (junction 658) -> (junction 659) [order 1] : [HandleIn > HandleOut]
    (junction 658) -> (junction 660) [order 2]
    (junction 659) -> (junction 661) : {HandleOut = HandleIn;}
    (junction 661) -> (junction 660)
    (junction 660) -> (junction 662)
  state ResetTransitionFlags [function]
    (default) -> (junction 669) : {DETERMINE_TAP_CHANGE = false;
        | DETERMINE_VLOCALBUS = false;
        | EXIT = false;
        | FINISHED = false;
        | GET_TEST_VALUES = false;
        | GET_VOLTAGE = false;
        | GET_VOLTAGEWLDC = false;
        | MAKE_TAP_CHANGE = false;
        | REV_NEUTRAL = false;}
  state WindingVoltages = GetWindingVoltages(Transformer, IndicatedWinding) [function]
    (default) -> (junction 674) : % Intend to store WindingVoltages in VBuffer
        | % Fills array with voltages across indicated winding
  state vt = ComputeVTerminal [function]
    (default) -> (junction 678) : % Iteration through order of admittance matrix
    (junction 679) -> (junction 677) [order 1] : [ii <= Yorder]
    (junction 677) -> (junction 680) : {vt(i) = NodeV(NodeRef(i));}
    (junction 678) -> (junction 679) : {ii = 1;}
    (junction 680) -> (junction 679) : {ii = ii + 1;}
    (junction 679) -> (junction 681) [order 2]
  state Result = GetControlVoltage [function]
    (default) -> (junction 689)
    (junction 689) -> (junction 690) [order 1] : [FPTphase == FPTphases.MAXPHASE]
        | % controlled phase is that with greatest |V|
    (junction 689) -> (junction 701) [order 2]
    (junction 690) -> (junction 692) : {ControlledPhase = 1;
        | % abs is equivalent to Cabs:
        | V = abs( VBuffer(ControlledPhase) );}
        | % Iteration through remaining phases:
    (junction 695) -> (junction 691) [order 1] : [ii <= Nphs]
    (junction 691) -> (junction 693)
    (junction 692) -> (junction 695) : {ii = 2;}
    (junction 693) -> (junction 694) [order 1] : [abs( VBuffer(ControlledPhase)) > V]
        | % if it's GREATER, make it the new V
    (junction 693) -> (junction 696) [order 2]
    (junction 694) -> (junction 697) : {V = VBuffer(ControlledPhase);
        | ControlledPhase = ii;}
    (junction 698) -> (junction 695) : {ii = ii+1;}
    (junction 695) -> (junction 700) [order 2]
    (junction 697) -> (junction 696)
    (junction 696) -> (junction 698) : {Result = VBuffer(FPTphase) / PTRatio;
        | % Complex divided by real
        | }
    (junction 700) -> (junction 699)
    (junction 699) -> (junction 711)
    (junction 701) -> (junction 702) [order 1] : [FPTphase == FPTphases.MINPHASE]
        | % controlled phase is that with least |V|
    (junction 702) -> (junction 704) : {ControlledPhase = 1;
        | % abs is equivalent to Cabs:
        | V = abs( VBuffer(ControlledPhase) );}
        | % Iteration through remaining phases:
    (junction 701) -> (junction 714) [order 2] : % just use one phase because
        | % that's what most controls do:
        | {Result = VBuffer(ControlledPhase) / PTRatio;
        | ControlledPhase = FPTphase;}
    (junction 707) -> (junction 703) [order 1] : [ii <= Nphs]
    (junction 703) -> (junction 705)
    (junction 704) -> (junction 707) : {ii = 2;}
    (junction 705) -> (junction 706) [order 1] : [abs( VBuffer(ControlledPhase)) < V]
        | % if it's LESS, make it the new V
    (junction 705) -> (junction 708) [order 2]
    (junction 706) -> (junction 709) : {V = VBuffer(ControlledPhase);
        | ControlledPhase = ii;}
    (junction 710) -> (junction 707) : {ii = ii+1;}
    (junction 707) -> (junction 712) [order 2]
    (junction 709) -> (junction 708)
    (junction 708) -> (junction 710) : {Result = VBuffer(FPTphase) / PTRatio;
        | % Complex divided by real
        | }
    (junction 712) -> (junction 711)
    (junction 711) -> (junction 713)
    (junction 713) -> (junction 714)
    (junction 714) -> (junction 715)
  state Result = ComputeTimeDelay(Vavg) [function]
    (default) -> (junction 751)
    (junction 751) -> (junction 752) [order 1] : [Finversetime]
    (junction 751) -> (junction 753) [order 2] : % determines which regulator control will act first,
        | % default is 15s
        | {Result = TimeDelay;}
    (junction 752) -> (junction 754) : % TimeDelay is adjusted inversely proportional to
        | % the amount that voltage is outside the band,
        | % down to 10 percent of specified time delay
        | % (Further out of band = band - 1> less time delay)
        | {Result = TimeDelay / min(10.0, 2.0*abs(Vreg - Vavg)/Bandwidth);}
    (junction 754) -> (junction 753)
    (junction 753) -> (junction 755)
  (default) -> ControlFlow
  data: CodeVal function_input double; DelayVal function_input double; h function_output double; Transformer function_input double; IndicatedWinding function_input double; WindingVoltages function_output double; vt function_output double; Result function_output double; Vavg function_input double; Result function_output double; Inputs input Bus: InputsBus; BandTest local double =0; BoostNeeded local double =0; ControlledTransformer local double; Increment local double =0; ReversePending local boolean =false; TapChangeIsNeeded local boolean =false; Vactual local double =0; Vboost local double =0; Vcontrol local double =0; Vlocalbus local double =0; VregTest local double =0; EPSILON local double =1.0e-12; R local double =0; X local double =0; BaseVoltage local double; CBuffer local double; ControlledElement local double; ControlledPhase local double; ElementTerminal local uint8 =1; Fnphases local double; InCogenMode local boolean =false; InReverseMode local boolean =false; LDCActive local boolean =false; LookingForward local boolean =false; MaxTap local double; MinTap local double; NodeV local double; PresentTap local double; RevPowerThreshold local double; ReverseNeutral local boolean =false; TapIncrement local double; TapWinding local uint8 =1; VBuffer local double; VlimitActive local boolean =false; Winding local double; revLDC_Z local double =0; revR local double =0; revX local double =0; TransformerConnection local int32 =0; VLDC local double =0; Vterminal local double; Bandwidth local double =3; CogenEnabled local boolean =false; FwdPower local double =0; ILDC local double =0; IsReversible local boolean =false; LDC_Z local double =0; PTRatio local double =60; RevBandwidth local double =3; RevVreg local double =120; TapLimitPerChange local uint8 =16; UsingRegulatedBus local boolean =false; Vlimit local double =0; Vreg local double =120; ControlAction output Enum: ActionCodes; Armed input boolean =false; TapChangeToMake local double; HandleOut output double =0; Delay output double =0; DoActions output Enum: QueueActions; RevBackHandle local uint8 =0; RevHandle output uint8 =0; REV_NEUTRAL local boolean =false; RevDelay local double; ControlledTransformerWindingVoltages local double; ControlledTransformerConnection local double; EXIT local boolean =false; FINISHED local boolean =false; GET_TEST_VALUES local boolean =false; MAKE_TAP_CHANGE local boolean =false; DETERMINE_TAP_CHANGE local boolean =false; GET_VOLTAGE local boolean =false; GET_VOLTAGEWLDC local boolean =false; DETERMINE_VLOCALBUS local boolean =false; TapDelay local double; HandleIn input double; PendingTapChange output double

== stateflow chart Action Coordinator ==
  state Asleep
  state SendingRegCtrlAction
    en:OutputAction.data = ...
    RegCtrlAction.data;
    send(OutputAction);
  state SendingSolverAction
    en:OutputAction.data = ...
    SolverAction.data;
    send(SolverAction);
  state SendingExecAction
    en:OutputAction.data = ...
    ExecAction.data;
    send(OutputAction);
  (default) -> Asleep
  Asleep -> SendingRegCtrlAction [order 1] : RegCtrlAction
  Asleep -> SendingSolverAction [order 3] : SolverAction
  SendingSolverAction -> Asleep
  SendingRegCtrlAction -> Asleep
  Asleep -> SendingExecAction [order 2] : ExecAction
  SendingExecAction -> Asleep
  data: RegCtrlAction input double; ExecAction input double; SolverAction input double; OutputAction output double
